simulink model "Regulation_01"  (R2022b)
settings: Solver=ode4  StartTime=0.0  StopTime=50  FixedStep=1e-3  MaxStep=1e-3  RelTol=1e-3
undefined symbols (not defined in the file or in its folder): p1, p2, p3, PR_kv, PR_kw, v_sat, w_sat, x_d, y_d
libraries: dspsigops x3
settings Model: Creator=david  LastModifiedBy=aless

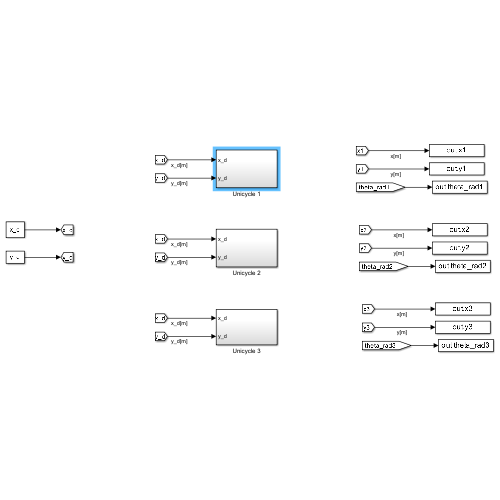
[thumbnail: Simulink's stored preview of the top-level diagram]
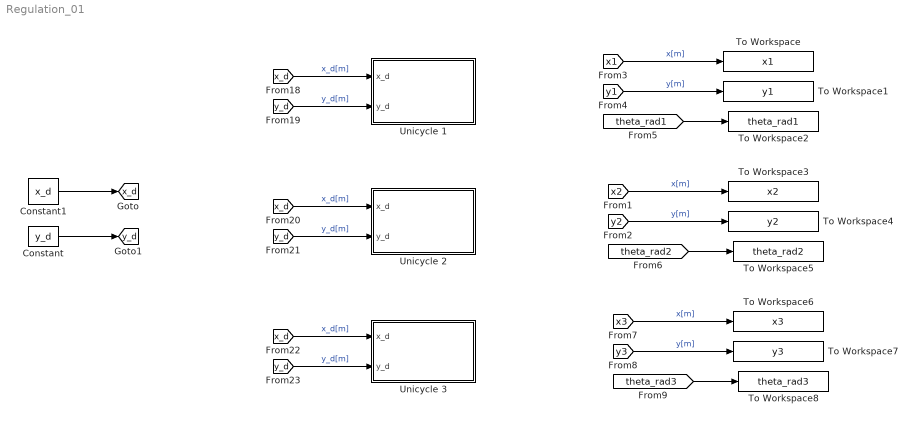
== system Regulation_01 ==
  Constant : Constant  Value=y_d
  Constant1 : Constant  Value=x_d
  To Workspace : ToWorkspace  VariableName=x1  SaveFormat=Structure With Time  SampleTime=-1
  To Workspace1 : ToWorkspace  VariableName=y1  SaveFormat=Structure With Time  SampleTime=-1
  To Workspace2 : ToWorkspace  VariableName=theta_rad1  SaveFormat=Structure With Time  SampleTime=-1
  To Workspace3 : ToWorkspace  VariableName=x2  SaveFormat=Structure With Time  SampleTime=-1
  To Workspace4 : ToWorkspace  VariableName=y2  SaveFormat=Structure With Time  SampleTime=-1
  To Workspace5 : ToWorkspace  VariableName=theta_rad2  SaveFormat=Structure With Time  SampleTime=-1
  To Workspace6 : ToWorkspace  VariableName=x3  SaveFormat=Structure With Time  SampleTime=-1
  To Workspace7 : ToWorkspace  VariableName=y3  SaveFormat=Structure With Time  SampleTime=-1
  To Workspace8 : ToWorkspace  VariableName=theta_rad3  SaveFormat=Structure With Time  SampleTime=-1
  Unicycle 1 : Subsystem
  Unicycle 2 : Subsystem
  Unicycle 3 : Subsystem
  tag scope: x_d=global, y_d=global
  wires:
  [x1] -> To Workspace/1  "x[m]"
  [y1] -> To Workspace1/1  "y[m]"
  [theta_rad1] -> To Workspace2/1
  [x2] -> To Workspace3/1  "x[m]"
  [y2] -> To Workspace4/1  "y[m]"
  [theta_rad2] -> To Workspace5/1
  [theta_rad3] -> To Workspace8/1
  [y3] -> To Workspace7/1  "y[m]"
  [x3] -> To Workspace6/1  "x[m]"
  Constant1/1 -> [x_d]
  Constant/1 -> [y_d]
  [x_d] -> Unicycle 1/1(x_d)  "x_d[m]"
  [y_d] -> Unicycle 1/2(y_d)  "y_d[m]"
  [y_d] -> Unicycle 2/2(y_d)  "y_d[m]"
  [x_d] -> Unicycle 2/1(x_d)  "x_d[m]"
  [y_d] -> Unicycle 3/2(y_d)  "y_d[m]"
  [x_d] -> Unicycle 3/1(x_d)  "x_d[m]"

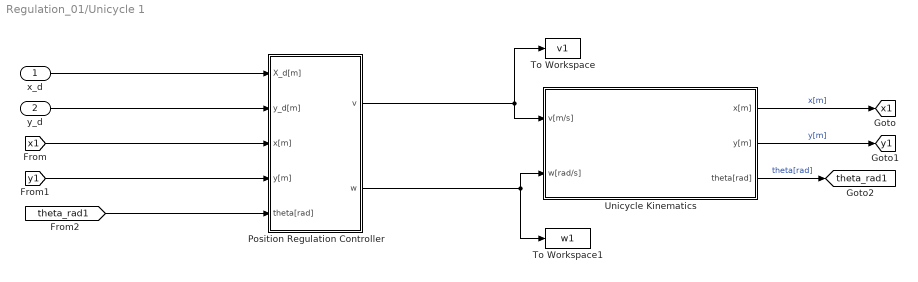
== system Regulation_01/Unicycle 1 ==
  x_d : Inport
  y_d : Inport  Port=2
  Position Regulation Controller : Subsystem
  To Workspace : ToWorkspace  VariableName=v1  SaveFormat=Structure With Time  SampleTime=-1
  To Workspace1 : ToWorkspace  VariableName=w1  SaveFormat=Structure With Time  SampleTime=-1
  Unicycle Kinematics : Subsystem
  tag scope: theta_rad1=global, x1=global, y1=global
  wires:
  Unicycle Kinematics/3(theta[rad]) -> [theta_rad1]  "theta[rad]"
  [y1] -> Position Regulation Controller/4(y[m])
  [theta_rad1] -> Position Regulation Controller/5(theta[rad])
  Unicycle Kinematics/2(y[m]) -> [y1]  "y[m]"
  [x1] -> Position Regulation Controller/3(x[m])
  Unicycle Kinematics/1(x[m]) -> [x1]  "x[m]"
  x_d/1 -> Position Regulation Controller/1(X_d[m])
  y_d/1 -> Position Regulation Controller/2(y_d[m])
  Position Regulation Controller/2(w) -> Unicycle Kinematics/2(w[rad/s]), To Workspace1/1
  Position Regulation Controller/1(v) -> Unicycle Kinematics/1(v[m/s]), To Workspace/1

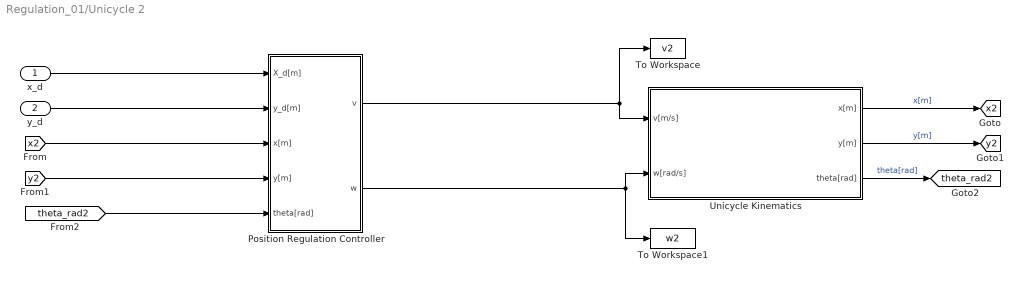
== system Regulation_01/Unicycle 2 ==
  x_d : Inport
  y_d : Inport  Port=2
  Position Regulation Controller : Subsystem
  To Workspace : ToWorkspace  VariableName=v2  SaveFormat=Structure With Time  SampleTime=-1
  To Workspace1 : ToWorkspace  VariableName=w2  SaveFormat=Structure With Time  SampleTime=-1
  Unicycle Kinematics : Subsystem
  tag scope: theta_rad2=global, x2=global, y2=global
  wires:
  Unicycle Kinematics/3(theta[rad]) -> [theta_rad2]  "theta[rad]"
  [y2] -> Position Regulation Controller/4(y[m])
  [theta_rad2] -> Position Regulation Controller/5(theta[rad])
  Unicycle Kinematics/2(y[m]) -> [y2]  "y[m]"
  [x2] -> Position Regulation Controller/3(x[m])
  Unicycle Kinematics/1(x[m]) -> [x2]  "x[m]"
  x_d/1 -> Position Regulation Controller/1(X_d[m])
  y_d/1 -> Position Regulation Controller/2(y_d[m])
  Position Regulation Controller/2(w) -> Unicycle Kinematics/2(w[rad/s]), To Workspace1/1
  Position Regulation Controller/1(v) -> Unicycle Kinematics/1(v[m/s]), To Workspace/1

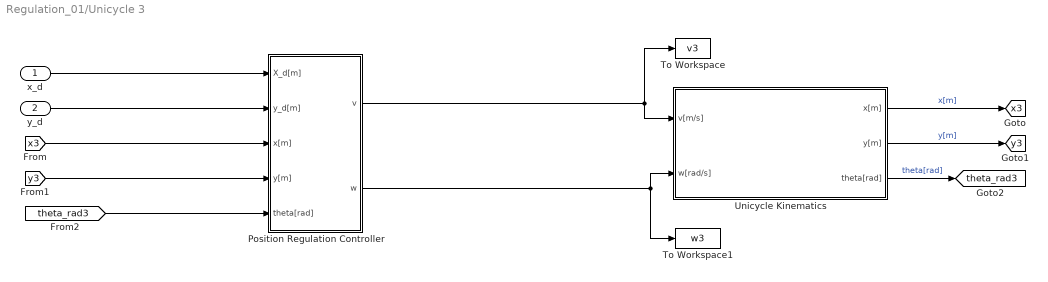
== system Regulation_01/Unicycle 3 ==
  x_d : Inport
  y_d : Inport  Port=2
  Position Regulation Controller : Subsystem
  To Workspace : ToWorkspace  VariableName=v3  SaveFormat=Structure With Time  SampleTime=-1
  To Workspace1 : ToWorkspace  VariableName=w3  SaveFormat=Structure With Time  SampleTime=-1
  Unicycle Kinematics : Subsystem
  tag scope: theta_rad3=global, x3=global, y3=global
  wires:
  Unicycle Kinematics/3(theta[rad]) -> [theta_rad3]  "theta[rad]"
  [y3] -> Position Regulation Controller/4(y[m])
  [theta_rad3] -> Position Regulation Controller/5(theta[rad])
  Unicycle Kinematics/2(y[m]) -> [y3]  "y[m]"
  [x3] -> Position Regulation Controller/3(x[m])
  Unicycle Kinematics/1(x[m]) -> [x3]  "x[m]"
  x_d/1 -> Position Regulation Controller/1(X_d[m])
  y_d/1 -> Position Regulation Controller/2(y_d[m])
  Position Regulation Controller/2(w) -> To Workspace1/1, Unicycle Kinematics/2(w[rad/s])
  Position Regulation Controller/1(v) -> Unicycle Kinematics/1(v[m/s]), To Workspace/1

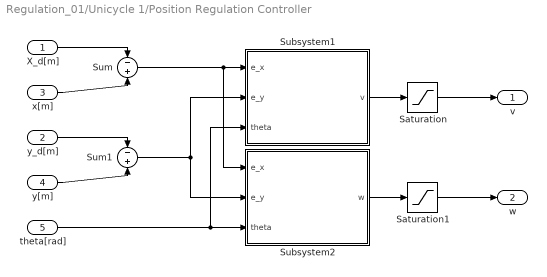
== system Regulation_01/Unicycle 1/Position Regulation Controller ==
  X_d[m] : Inport
  y_d[m] : Inport  Port=2
  x[m] : Inport  Port=3
  y[m] : Inport  Port=4
  theta[rad] : Inport  Port=5
  Saturation : Saturate  UpperLimit=v_sat  LowerLimit=-v_sat
  Saturation1 : Saturate  UpperLimit=w_sat  LowerLimit=-w_sat
  Subsystem1 : Subsystem
  Subsystem2 : Subsystem
  Sum : Sum  Inputs=-+
  Sum1 : Sum  Inputs=-+
  v : Outport
  w : Outport  Port=2
  wires:
  X_d[m]/1 -> Sum/1
  x[m]/1 -> Sum/2
  y_d[m]/1 -> Sum1/1
  y[m]/1 -> Sum1/2
  theta[rad]/1 -> Subsystem2/3(theta), Subsystem1/3(theta)
  Sum/1 -> Subsystem2/1(e_x), Subsystem1/1(e_x)
  Sum1/1 -> Subsystem1/2(e_y), Subsystem2/2(e_y)
  Subsystem2/1(w) -> Saturation1/1
  Subsystem1/1(v) -> Saturation/1
  Saturation/1 -> v/1
  Saturation1/1 -> w/1

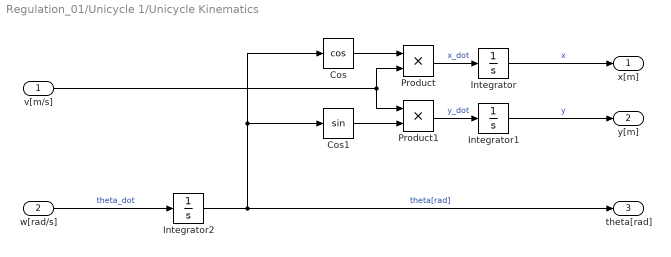
== system Regulation_01/Unicycle 1/Unicycle Kinematics ==
  v[m/s] : Inport
  w[rad/s] : Inport  Port=2
  Cos : Trigonometry  Operator=cos
  Cos1 : Trigonometry
  Integrator : Integrator  InitialCondition=p1(1)
  Integrator1 : Integrator  InitialCondition=p1(2)
  Integrator2 : Integrator  InitialCondition=p1(3)
  Product : Product
  Product1 : Product
  x[m] : Outport
  y[m] : Outport  Port=2
  theta[rad] : Outport  Port=3
  wires:
  Integrator/1 -> x[m]/1  "x"
  Integrator1/1 -> y[m]/1  "y"
  w[rad/s]/1 -> Integrator2/1  "theta_dot"
  Integrator2/1 -> Cos/1, Cos1/1, theta[rad]/1  "theta[rad]"
  Product/1 -> Integrator/1  "x_dot"
  Cos1/1 -> Product1/2
  Cos/1 -> Product/1
  v[m/s]/1 -> Product1/1, Product/2
  Product1/1 -> Integrator1/1  "y_dot"

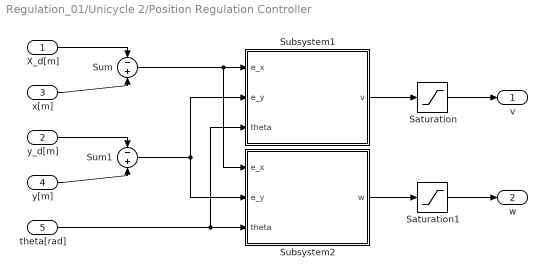
== system Regulation_01/Unicycle 2/Position Regulation Controller ==
  X_d[m] : Inport
  y_d[m] : Inport  Port=2
  x[m] : Inport  Port=3
  y[m] : Inport  Port=4
  theta[rad] : Inport  Port=5
  Saturation : Saturate  UpperLimit=v_sat  LowerLimit=-v_sat
  Saturation1 : Saturate  UpperLimit=w_sat  LowerLimit=-w_sat
  Subsystem1 : Subsystem
  Subsystem2 : Subsystem
  Sum : Sum  Inputs=-+
  Sum1 : Sum  Inputs=-+
  v : Outport
  w : Outport  Port=2
  wires:
  X_d[m]/1 -> Sum/1
  x[m]/1 -> Sum/2
  y_d[m]/1 -> Sum1/1
  y[m]/1 -> Sum1/2
  theta[rad]/1 -> Subsystem2/3(theta), Subsystem1/3(theta)
  Sum/1 -> Subsystem2/1(e_x), Subsystem1/1(e_x)
  Sum1/1 -> Subsystem1/2(e_y), Subsystem2/2(e_y)
  Subsystem2/1(w) -> Saturation1/1
  Subsystem1/1(v) -> Saturation/1
  Saturation/1 -> v/1
  Saturation1/1 -> w/1

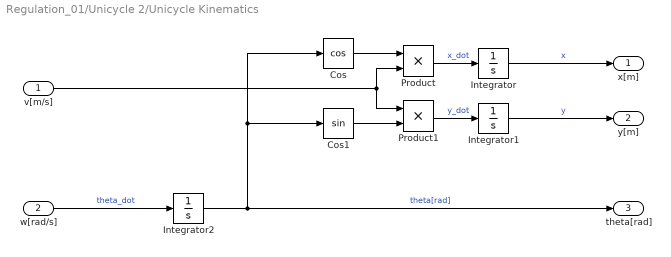
== system Regulation_01/Unicycle 2/Unicycle Kinematics ==
  v[m/s] : Inport
  w[rad/s] : Inport  Port=2
  Cos : Trigonometry  Operator=cos
  Cos1 : Trigonometry
  Integrator : Integrator  InitialCondition=p2(1)
  Integrator1 : Integrator  InitialCondition=p2(2)
  Integrator2 : Integrator  InitialCondition=p2(3)
  Product : Product
  Product1 : Product
  x[m] : Outport
  y[m] : Outport  Port=2
  theta[rad] : Outport  Port=3
  wires:
  Integrator/1 -> x[m]/1  "x"
  Integrator1/1 -> y[m]/1  "y"
  w[rad/s]/1 -> Integrator2/1  "theta_dot"
  Integrator2/1 -> Cos/1, Cos1/1, theta[rad]/1  "theta[rad]"
  Product/1 -> Integrator/1  "x_dot"
  Cos1/1 -> Product1/2
  Cos/1 -> Product/1
  v[m/s]/1 -> Product1/1, Product/2
  Product1/1 -> Integrator1/1  "y_dot"

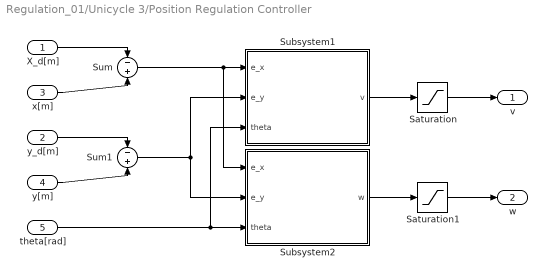
== system Regulation_01/Unicycle 3/Position Regulation Controller ==
  X_d[m] : Inport
  y_d[m] : Inport  Port=2
  x[m] : Inport  Port=3
  y[m] : Inport  Port=4
  theta[rad] : Inport  Port=5
  Saturation : Saturate  UpperLimit=v_sat  LowerLimit=-v_sat
  Saturation1 : Saturate  UpperLimit=w_sat  LowerLimit=-w_sat
  Subsystem1 : Subsystem
  Subsystem2 : Subsystem
  Sum : Sum  Inputs=-+
  Sum1 : Sum  Inputs=-+
  v : Outport
  w : Outport  Port=2
  wires:
  X_d[m]/1 -> Sum/1
  x[m]/1 -> Sum/2
  y_d[m]/1 -> Sum1/1
  y[m]/1 -> Sum1/2
  theta[rad]/1 -> Subsystem2/3(theta), Subsystem1/3(theta)
  Sum/1 -> Subsystem2/1(e_x), Subsystem1/1(e_x)
  Sum1/1 -> Subsystem1/2(e_y), Subsystem2/2(e_y)
  Subsystem2/1(w) -> Saturation1/1
  Subsystem1/1(v) -> Saturation/1
  Saturation/1 -> v/1
  Saturation1/1 -> w/1

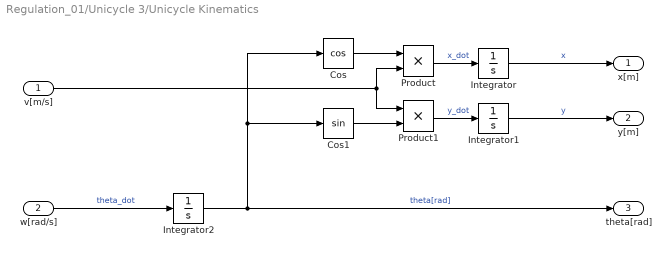
== system Regulation_01/Unicycle 3/Unicycle Kinematics ==
  v[m/s] : Inport
  w[rad/s] : Inport  Port=2
  Cos : Trigonometry  Operator=cos
  Cos1 : Trigonometry
  Integrator : Integrator  InitialCondition=p3(1)
  Integrator1 : Integrator  InitialCondition=p3(2)
  Integrator2 : Integrator  InitialCondition=p3(3)
  Product : Product
  Product1 : Product
  x[m] : Outport
  y[m] : Outport  Port=2
  theta[rad] : Outport  Port=3
  wires:
  Integrator/1 -> x[m]/1  "x"
  Integrator1/1 -> y[m]/1  "y"
  w[rad/s]/1 -> Integrator2/1  "theta_dot"
  Integrator2/1 -> Cos/1, Cos1/1, theta[rad]/1  "theta[rad]"
  Product/1 -> Integrator/1  "x_dot"
  Cos1/1 -> Product1/2
  Cos/1 -> Product/1
  v[m/s]/1 -> Product1/1, Product/2
  Product1/1 -> Integrator1/1  "y_dot"

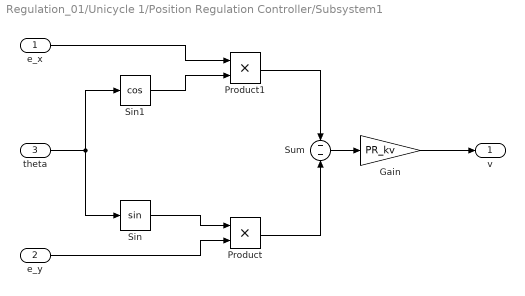
== system Regulation_01/Unicycle 1/Position Regulation Controller/Subsystem1 ==
  e_x : Inport
  e_y : Inport  Port=2
  theta : Inport  Port=3
  Gain : Gain  Gain=PR_kv
  Product : Product
  Product1 : Product
  Sin : Trigonometry
  Sin1 : Trigonometry  Operator=cos
  Sum : Sum  Inputs=--
  v : Outport
  wires:
  e_y/1 -> Product/2
  theta/1 -> Sin/1, Sin1/1
  Sum/1 -> Gain/1
  Gain/1 -> v/1
  Sin/1 -> Product/1
  Product/1 -> Sum/2
  e_x/1 -> Product1/1
  Sin1/1 -> Product1/2
  Product1/1 -> Sum/1

== system Regulation_01/Unicycle 1/Position Regulation Controller/Subsystem2 ==
  e_x : Inport
  e_y : Inport  Port=2
  theta : Inport  Port=3
  Atan2 : Trigonometry  Operator=atan2  ApproximationMethod=Lookup  NumberOfDataPoints=2
  Constant : Constant  Value=pi
  Gain : Gain  Gain=PR_kw
  Sum : Sum  Inputs=+-+
  Unwrap : dspsigops/Unwrap  tol=pi  InputProcessing=Columns as channels (frame based)  running=off
  w : Outport
  wires:
  e_x/1 -> Atan2/2
  e_y/1 -> Atan2/1
  theta/1 -> Sum/2
  Sum/1 -> Gain/1
  Atan2/1 -> Unwrap/1
  Constant/1 -> Sum/3
  Gain/1 -> w/1
  Unwrap/1 -> Sum/1

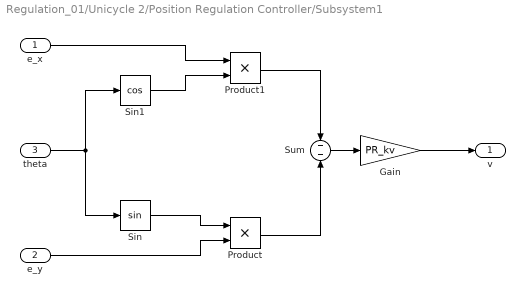
== system Regulation_01/Unicycle 2/Position Regulation Controller/Subsystem1 ==
  e_x : Inport
  e_y : Inport  Port=2
  theta : Inport  Port=3
  Gain : Gain  Gain=PR_kv
  Product : Product
  Product1 : Product
  Sin : Trigonometry
  Sin1 : Trigonometry  Operator=cos
  Sum : Sum  Inputs=--
  v : Outport
  wires:
  e_y/1 -> Product/2
  theta/1 -> Sin/1, Sin1/1
  Sum/1 -> Gain/1
  Gain/1 -> v/1
  Sin/1 -> Product/1
  Product/1 -> Sum/2
  e_x/1 -> Product1/1
  Sin1/1 -> Product1/2
  Product1/1 -> Sum/1

== system Regulation_01/Unicycle 2/Position Regulation Controller/Subsystem2 ==
  e_x : Inport
  e_y : Inport  Port=2
  theta : Inport  Port=3
  Atan2 : Trigonometry  Operator=atan2  ApproximationMethod=Lookup  NumberOfDataPoints=2
  Constant : Constant  Value=pi
  Gain : Gain  Gain=PR_kw
  Sum : Sum  Inputs=+-+
  Unwrap : dspsigops/Unwrap  tol=pi  InputProcessing=Columns as channels (frame based)  running=off
  w : Outport
  wires:
  e_x/1 -> Atan2/2
  e_y/1 -> Atan2/1
  theta/1 -> Sum/2
  Sum/1 -> Gain/1
  Atan2/1 -> Unwrap/1
  Constant/1 -> Sum/3
  Gain/1 -> w/1
  Unwrap/1 -> Sum/1

== system Regulation_01/Unicycle 3/Position Regulation Controller/Subsystem1 ==
  e_x : Inport
  e_y : Inport  Port=2
  theta : Inport  Port=3
  Gain : Gain  Gain=PR_kv
  Product : Product
  Product1 : Product
  Sin : Trigonometry
  Sin1 : Trigonometry  Operator=cos
  Sum : Sum  Inputs=--
  v : Outport
  wires:
  e_y/1 -> Product/2
  theta/1 -> Sin/1, Sin1/1
  Sum/1 -> Gain/1
  Gain/1 -> v/1
  Sin/1 -> Product/1
  Product/1 -> Sum/2
  e_x/1 -> Product1/1
  Sin1/1 -> Product1/2
  Product1/1 -> Sum/1

== system Regulation_01/Unicycle 3/Position Regulation Controller/Subsystem2 ==
  e_x : Inport
  e_y : Inport  Port=2
  theta : Inport  Port=3
  Atan2 : Trigonometry  Operator=atan2  ApproximationMethod=Lookup  NumberOfDataPoints=2
  Constant : Constant  Value=pi
  Gain : Gain  Gain=PR_kw
  Sum : Sum  Inputs=+-+
  Unwrap : dspsigops/Unwrap  tol=pi  InputProcessing=Columns as channels (frame based)  running=off
  w : Outport
  wires:
  e_x/1 -> Atan2/2
  e_y/1 -> Atan2/1
  theta/1 -> Sum/2
  Sum/1 -> Gain/1
  Atan2/1 -> Unwrap/1
  Constant/1 -> Sum/3
  Gain/1 -> w/1
  Unwrap/1 -> Sum/1
